simulink model "untitled"  (R2022a)
settings: Solver=VariableStepAuto  StartTime=0.0  StopTime=30.0  RelTol=1e-3
libraries: commanapbnd3 x2, commrandsrc3 x1
settings Model: Creator=ma  LastModifiedBy=ma

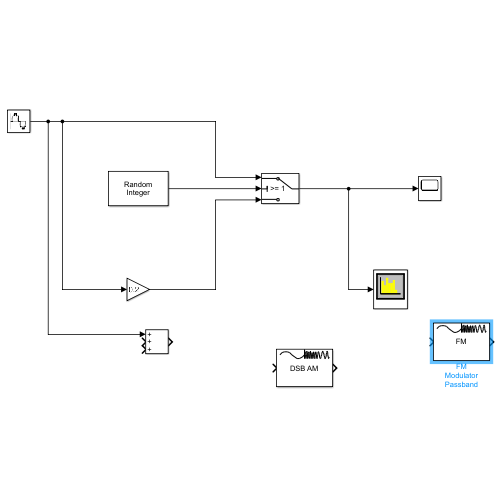
[thumbnail: Simulink's stored preview of the top-level diagram]
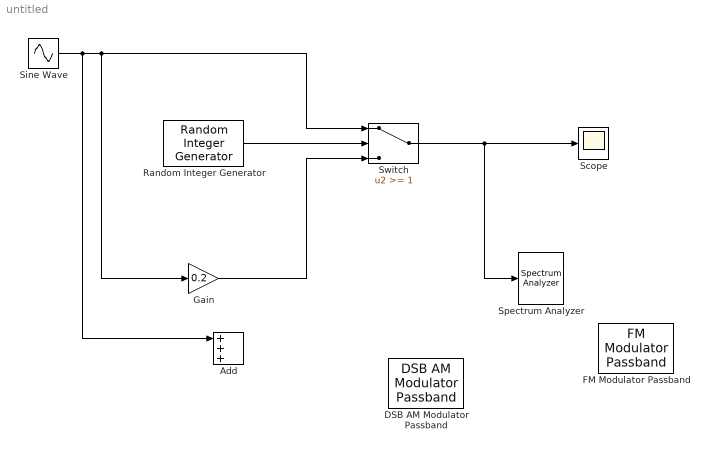
== system untitled ==
  Add : Sum  Inputs=+++
  DSB AM Modulator Passband : commanapbnd3/DSB AM Modulator Passband  Fc=300  Ph=0  Offset=1
      settings: SourceProductBaseCode=CM
  FM Modulator Passband : commanapbnd3/FM Modulator Passband  Fc=300  Ph=0  Kc=50
      settings: SourceProductBaseCode=CM
  Gain : Gain  Gain=0.2
  Random Integer Generator : commrandsrc3/Random Integer Generator  SetSize=2  SeedSource=Parameter  Seed=50  SampleTime=1  SamplesPerFrame=1  OutputDataType=double  SimulateUsing=Interpreted execution
  Scope : Scope
  Sine Wave : Sin  Frequency=2*pi*10  SampleTime=1/100
  Spectrum Analyzer : SpectrumAnalyzer
  Switch : Switch  Threshold=1  SaturateOnIntegerOverflow=off  InputSameDT=off
  wires:
  Random Integer Generator/1 -> Switch/2
  Switch/1 -> Spectrum Analyzer/1, Scope/1
  Gain/1 -> Switch/3
  Sine Wave/1 -> Add/1, Switch/1, Gain/1
